simulink model "lab3_1"  (R2022a)
settings: Solver=FixedStepAuto  StartTime=0.0  StopTime=Tmdl  FixedStep=To/100  RelTol=1e-3
undefined symbols (not defined in the file or in its folder): an, dsc, To
settings Model: Creator=Professional  LastModifiedBy=osini

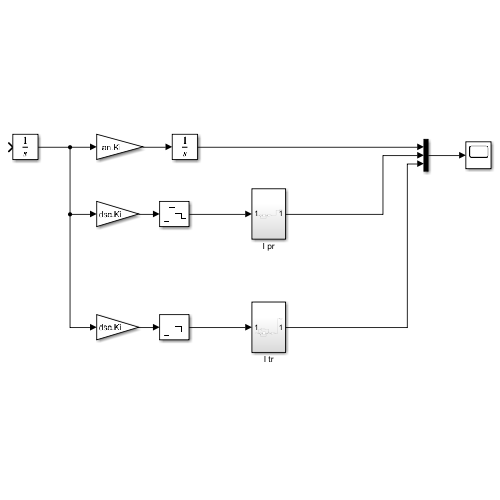
[thumbnail: Simulink's stored preview of the top-level diagram]
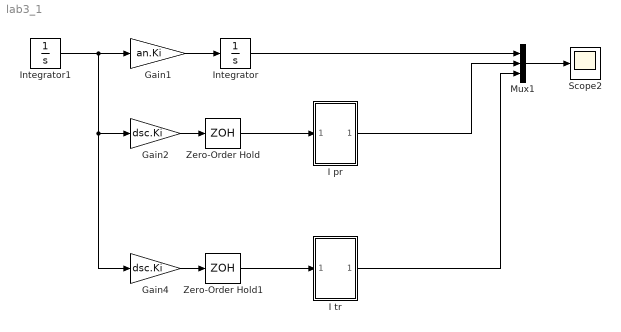
== system lab3_1 ==
  Gain1 : Gain  Gain=an.Ki
  Gain2 : Gain  Gain=dsc.Ki
  Gain4 : Gain  Gain=dsc.Ki
  I pr : Subsystem
  I tr : Subsystem
  Integrator : Integrator
  Integrator1 : Integrator  InitialCondition=1
  Mux1 : Mux  Inputs=3
  Scope2 : Scope
  Zero-Order Hold : ZeroOrderHold  SampleTime=To
  Zero-Order Hold1 : ZeroOrderHold  SampleTime=To
  wires:
  Gain1/1 -> Integrator/1
  Mux1/1 -> Scope2/1
  Gain2/1 -> Zero-Order Hold/1
  Integrator/1 -> Mux1/1
  Gain4/1 -> Zero-Order Hold1/1
  Integrator1/1 -> Gain4/1, Gain2/1, Gain1/1
  Zero-Order Hold/1 -> I pr/1(In1)
  I pr/1(Out1) -> Mux1/2
  Zero-Order Hold1/1 -> I tr/1(In1)
  I tr/1(Out1) -> Mux1/3

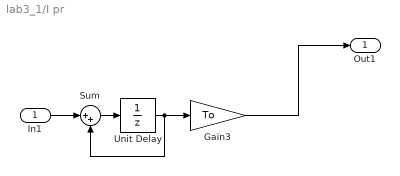
== system lab3_1/I pr ==
  In1 : Inport
  Gain3 : Gain  Gain=To
  Sum : Sum  Inputs=|++
  Unit Delay : UnitDelay  SampleTime=-1  HasFrameUpgradeWarning=on
  Out1 : Outport
  wires:
  Sum/1 -> Unit Delay/1
  Unit Delay/1 -> Sum/2, Gain3/1
  Gain3/1 -> Out1/1
  In1/1 -> Sum/1

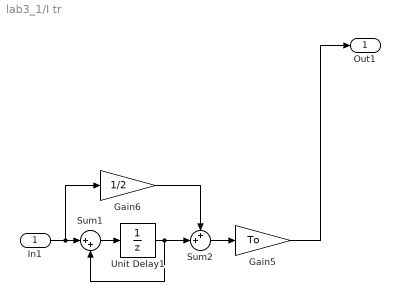
== system lab3_1/I tr ==
  In1 : Inport
  Gain5 : Gain  Gain=To
  Gain6 : Gain  Gain=1/2
  Sum1 : Sum  Inputs=|++
  Sum2 : Sum  Inputs=++|
  Unit Delay1 : UnitDelay  SampleTime=-1  HasFrameUpgradeWarning=on
  Out1 : Outport
  wires:
  In1/1 -> Gain6/1, Sum1/1
  Sum2/1 -> Gain5/1
  Sum1/1 -> Unit Delay1/1
  Gain5/1 -> Out1/1
  Unit Delay1/1 -> Sum2/2, Sum1/2
  Gain6/1 -> Sum2/1
